simulink model "PID_control"  (R2022a)
settings: Solver=ode3  StartTime=0.0  StopTime=inf  FixedStep=0.005  RelTol=1e-3
undefined symbols (not defined in the file): Angular, Linear
libraries: robotlib x7, robotcorelib x1
settings Model: Creator=Ronak Jain  LastModifiedBy=Ronak Jain
settings OptimizationCC: EnhancedBackFolding=on  PassReuseOutputArgsAs=Individual arguments  LifeSpan=inf  MaxStackSize=64  OptimizeBlockOrder=speed  DifferentSizesBufferReuse=on  OptimizationCustomize=off  EfficientTunableParamExpr=on
settings DebuggingCC: ParameterTunabilityLossMsg=error  BusObjectLabelMismatch=error
settings HardwareCC: ProdBitPerPointer=32  ProdBitPerSizeT=32  ProdBitPerPtrDiffT=32  ProdLargestAtomicFloat=None  ProdIntDivRoundTo=Undefined  ProdEndianess=Unspecified  ProdWordSize=32  ProdHWDeviceType=Generic->Unspecified (assume 32-bit Generic)  TargetBitPerPointer=64  TargetBitPerSizeT=64  TargetBitPerPtrDiffT=64  TargetLongLongMode=on  TargetIntDivRoundTo=Zero  TargetEndianess=LittleEndian  TargetWordSize=64  TargetHWDeviceType=MATLAB Host  ProdEqTarget=off
settings RTWCC: SystemTargetFile=ert.tlc  HardwareBoard=Robot Operating System (ROS)  TLCOptions="-aInlineSetEventsForThisBaseRateFcn=TLC_FALSE -aSuppressMultiTaskScheduler=TLC_FALSE  -aRateBasedStepFcn=0"  TemplateMakefile=ert_default_tmf  Toolchain=Catkin  TargetLang=C++
settings CodeAppCC: ForceParamTrailComments=on  IgnoreCustomStorageClasses=off  OperatorAnnotations=on  SimulinkDataObjDesc=on  SFDataObjDesc=on  InsertBlockDesc=on
settings ERTTargetCC: CodeInterfacePackaging=Reusable function  SupportContinuousTime=on  SupportVariableSizeSignals=on  ModelStepFunctionPrototypeControlCompliant=off  GenerateAllocFcn=on  MultiInstanceErrorCode=None  RootIOFormat=Part of model data structure

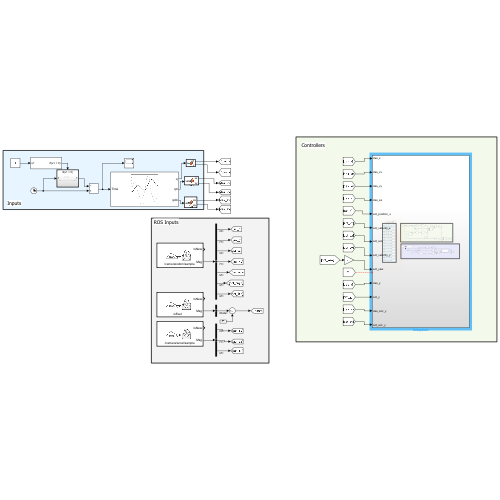
[thumbnail: Simulink's stored preview of the top-level diagram]
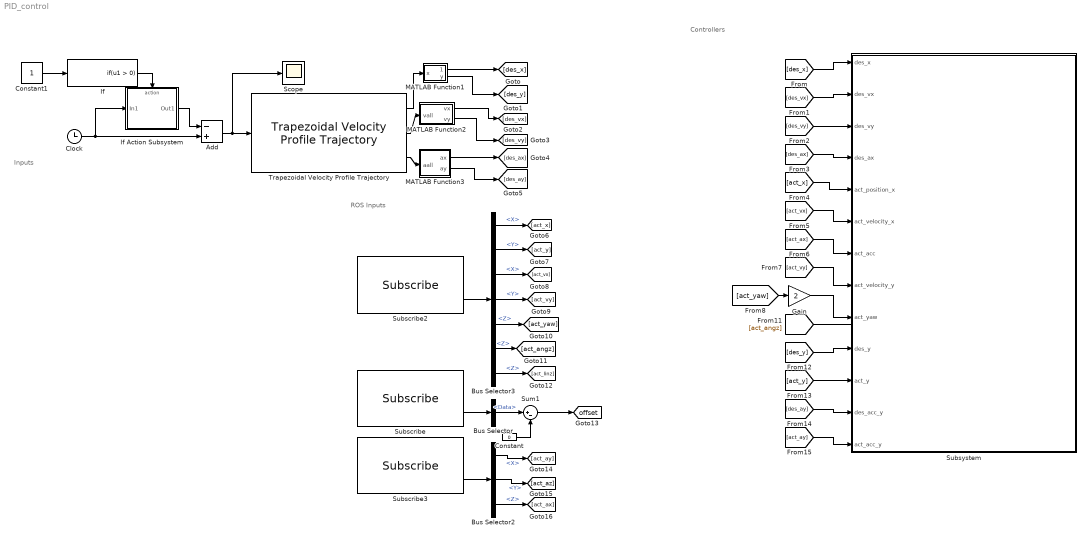
== system PID_control ==
  note: Inputs
  note: ROS Inputs
  note: Controllers
  Add : Sum  Inputs=-+
  Bus Selector : BusSelector  OutputSignals=Data
  Bus Selector2 : BusSelector  OutputSignals=LinearAcceleration.X,LinearAcceleration.Y,LinearAcceleration.Z
  Bus Selector3 : BusSelector  OutputSignals=Pose.Pose.Position.X,Pose.Pose.Position.Y,Twist.Twist.Linear.X,Twist.Twist.Linear.Y,Pose.Pose.Orientation.Z,Twist.Twist.Angular.Z,Twist.Twist.Linear.Z
  Clock : Clock
  Constant : Constant  Value=0
  Constant1 : Constant  SampleTime=-1
  Gain : Gain  Gain=2
  If : If  ShowElse=off
  If Action Subsystem : Subsystem  TreatAsAtomicUnit=on
  MATLAB Function1 : MATLAB Function  TreatAsAtomicUnit=on
  MATLAB Function2 : MATLAB Function  TreatAsAtomicUnit=on
  MATLAB Function3 : MATLAB Function  TreatAsAtomicUnit=on
  Scope : Scope
  Subscribe : robotlib/Subscribe  topicSource=Select from ROS network  topic=/offset  messageType=std_msgs/Float32  SampleTime=-1  legacyBusStruct=off  messageQueueLength=1
  Subscribe2 : robotlib/Subscribe  topicSource=Select from ROS network  topic=/camera/odom/sample  messageType=nav_msgs/Odometry  SampleTime=-1  legacyBusStruct=off  messageQueueLength=1
  Subscribe3 : robotlib/Subscribe  topicSource=Select from ROS network  topic=/camera/accel/sample  messageType=sensor_msgs/Imu  SampleTime=-1  legacyBusStruct=off  messageQueueLength=1
  Subsystem : Subsystem
  Sum1 : Sum  Inputs=|+-
  Trapezoidal Velocity Profile Trajectory : robotcorelib/Trapezoidal Velocity Profile Trajectory  WaypointSource=Internal  Waypoints=[0,2.5*3;0,0]  NumParams=2  Parameter1=Acceleration Time  Parameter2=End Time  ParameterSource=Internal  PeakVelocity=[ 2; 2 ]  Acceleration=[ 1; 2 ]  EndTime=[ 35*3;35*3]  AccelTime=[ 10; 10 ]  SimulateUsing=Interpreted execution
      settings: SourceProductBaseCode=RO,NV,RR,UV
  tag scope: offset=global
  wires:
  Subscribe3/2 -> Bus Selector2/1
  Trapezoidal Velocity Profile Trajectory/1 -> MATLAB Function1/1(x)
  If Action Subsystem/1(Out1) -> Add/1
  Subscribe2/2 -> Bus Selector3/1
  Subscribe/2 -> Bus Selector/1
  If/1 -> If Action Subsystem/Action
  Trapezoidal Velocity Profile Trajectory/2 -> MATLAB Function2/1(vall)
  Trapezoidal Velocity Profile Trajectory/3 -> MATLAB Function3/1(aall)
  Constant1/1 -> If/1
  Clock/1 -> Add/2, If Action Subsystem/1(In1)
  Add/1 -> Scope/1, Trapezoidal Velocity Profile Trajectory/1
  MATLAB Function1/1(x1) -> [des_x]
  MATLAB Function1/2(y) -> [des_y]
  MATLAB Function2/1(vx) -> [des_vx]
  MATLAB Function2/2(vy) -> [des_vy]
  MATLAB Function3/1(ax) -> [des_ax]
  MATLAB Function3/2(ay) -> [des_ay]
  Bus Selector3/1 -> [act_x]  "<X>"
  Bus Selector3/2 -> [act_y]  "<Y>"
  Bus Selector3/3 -> [act_vx]  "<X>"
  Bus Selector3/4 -> [act_vy]  "<Y>"
  Bus Selector3/5 -> [act_yaw]  "<Z>"
  Bus Selector3/6 -> [act_angz]  "<Z>"
  Bus Selector3/7 -> [act_linz]  "<Z>"
  Bus Selector2/1 -> [act_ay]  "<X>"
  Bus Selector2/2 -> [act_az]  "<Y>"
  Bus Selector2/3 -> [act_ax]  "<Z>"
  [des_x] -> Subsystem/1(des_x)
  [des_vx] -> Subsystem/2(des_vx)
  [des_vy] -> Subsystem/3(des_vy)
  [des_ax] -> Subsystem/4(des_ax)
  [act_x] -> Subsystem/5(act_position_x)
  [act_vx] -> Subsystem/6(act_velocity_x)
  [act_ax] -> Subsystem/7(act_acc)
  [act_vy] -> Subsystem/8(act_velocity_y)
  [act_yaw] -> Gain/1
  [act_angz] -> ?
  [des_y] -> Subsystem/10(des_y)
  [act_y] -> Subsystem/11(act_y)
  [des_ay] -> Subsystem/12(des_acc_y)
  [act_ay] -> Subsystem/13(act_acc_y)
  Gain/1 -> Subsystem/9(act_yaw)
  Bus Selector/1 -> Sum1/1  "<Data>"
  Sum1/1 -> [offset]
  Constant/1 -> Sum1/2

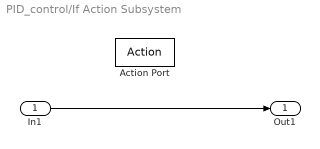
== system PID_control/If Action Subsystem ==
  In1 : Inport
  Action Port : ActionPort  PropagateVarSize=During execution  ActionPortLabel=if(u1 > 0)
  Out1 : Outport
  wires:
  In1/1 -> Out1/1

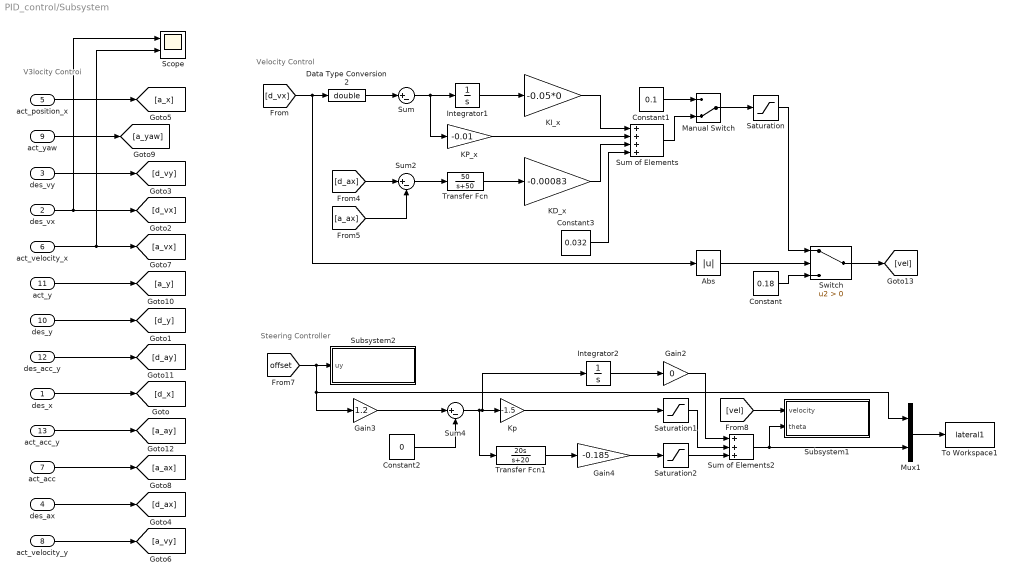
== system PID_control/Subsystem ==
  note: Velocity Control
  note: V3locity Controi
  note: Steering Controller
  des_x : Inport
  des_vx : Inport  Port=2
  des_vy : Inport  Port=3
  des_ax : Inport  Port=4
  act_position_x : Inport  Port=5
  act_velocity_x : Inport  Port=6
  act_acc : Inport  Port=7
  act_velocity_y : Inport  Port=8
  act_yaw : Inport  Port=9
  des_y : Inport  Port=10
  act_y : Inport  Port=11
  des_acc_y : Inport  Port=12
  act_acc_y : Inport  Port=13
  Abs : Abs  SaturateOnIntegerOverflow=off
  Constant : Constant  Value=0.18
  Constant1 : Constant  Value=0.1
  Constant2 : Constant  Value=0
  Constant3 : Constant  Value=0.032
  Data Type Conversion2 : DataTypeConversion  OutDataTypeStr=double  SaturateOnIntegerOverflow=off  RndMeth=Floor
  Gain2 : Gain  Gain=0
  Gain3 : Gain  Gain=1.2
  Gain4 : Gain  Gain=-0.185
  Integrator1 : Integrator
  Integrator2 : Integrator
  KD_x : Gain  Gain=-0.00083
  KI_x : Gain  Gain=-0.05*0
  KP_x : Gain  Gain=-0.01
  Kp : Gain  Gain=-1.5
  Manual Switch : ManualSwitch  CurrentSetting=0
  Mux1 : Mux  Inputs=2
  Saturation : Saturate  LowerLimit=-0.2
  Saturation1 : Saturate  UpperLimit=0.7  LowerLimit=-0.7
  Saturation2 : Saturate  UpperLimit=0.7  LowerLimit=-0.7
  Scope : Scope  NumInputPorts=2
  Subsystem1 : Subsystem
  Subsystem2 : Subsystem
  Sum : Sum  Inputs=|+-
  Sum of Elements : Sum  Inputs=++++
  Sum of Elements2 : Sum  Inputs=+++
  Sum2 : Sum  Inputs=|+-
  Sum4 : Sum  Inputs=|+-
  Switch : Switch  Criteria=u2 > Threshold  SaturateOnIntegerOverflow=off  InputSameDT=off
  To Workspace1 : ToWorkspace  VariableName=lateral1  SaveFormat=Timeseries  SampleTime=-1
  Transfer Fcn : TransferFcn  Numerator=[50]  Denominator=[1 50]
  Transfer Fcn1 : TransferFcn  Numerator=[20 0]  Denominator=[1 20]
  wires:
  KD_x/1 -> Sum of Elements/3
  Abs/1 -> Switch/2
  des_vx/1 -> Scope/1, [d_vx]
  des_vy/1 -> [d_vy]
  Constant/1 -> Switch/3
  Transfer Fcn/1 -> KD_x/1
  Manual Switch/1 -> Saturation/1
  Switch/1 -> [vel]
  Sum of Elements/1 -> Manual Switch/2
  Saturation/1 -> Switch/1
  Constant1/1 -> Manual Switch/1
  Constant3/1 -> Sum of Elements/4
  [a_ax] -> Sum2/2
  [d_ax] -> Sum2/1
  Sum2/1 -> Transfer Fcn/1
  KI_x/1 -> Sum of Elements/1
  Integrator1/1 -> KI_x/1
  act_velocity_y/1 -> [a_vy]
  act_yaw/1 -> [a_yaw]
  KP_x/1 -> Sum of Elements/2
  Data Type Conversion2/1 -> Sum/1
  Sum/1 -> KP_x/1, Integrator1/1
  des_x/1 -> [d_x]
  [d_vx] -> Data Type Conversion2/1, Abs/1
  des_acc_y/1 -> [d_ay]
  act_acc_y/1 -> [a_ay]
  des_y/1 -> [d_y]
  act_y/1 -> [a_y]
  act_velocity_x/1 -> Scope/2, [a_vx]
  act_acc/1 -> [a_ax]
  des_ax/1 -> [d_ax]
  act_position_x/1 -> [a_x]
  [offset] -> Mux1/1, Gain3/1, Subsystem2/1(uy)
  Gain2/1 -> Sum of Elements2/1
  Sum4/1 -> Kp/1, Integrator2/1, Transfer Fcn1/1
  [vel] -> Subsystem1/1(velocity)
  Sum of Elements2/1 -> Mux1/2, Subsystem1/2(theta)
  Constant2/1 -> Sum4/2
  Transfer Fcn1/1 -> Gain4/1
  Saturation1/1 -> Sum of Elements2/2
  Mux1/1 -> To Workspace1/1
  Integrator2/1 -> Gain2/1
  Gain3/1 -> Sum4/1
  Saturation2/1 -> Sum of Elements2/3
  Kp/1 -> Saturation1/1
  Gain4/1 -> Saturation2/1

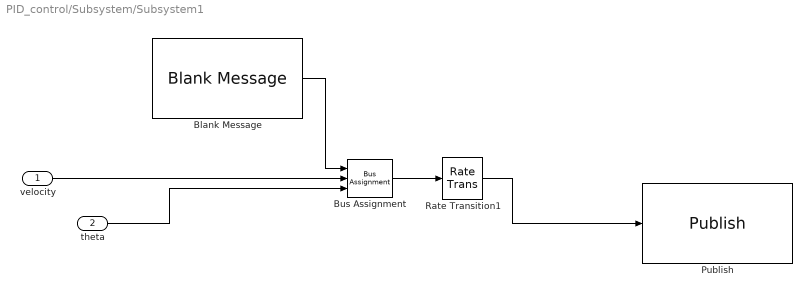
== system PID_control/Subsystem/Subsystem1 ==
  velocity : Inport
  theta : Inport  Port=2
  Blank Message : robotlib/Blank Message  messageClass=Message  entityType=geometry_msgs/Twist  messageType=geometry_msgs/Twist  SampleTime=-1  legacyBusStruct=off
  Bus Assignment : BusAssignment  AssignedSignals=Linear.X,Angular.Z
  Publish : robotlib/Publish  topicSource=Specify your own  topic=/move_velocity  messageType=geometry_msgs/Twist  legacyBusStruct=off  messageQueueLength=1
  Rate Transition1 : RateTransition
  wires:
  theta/1 -> Bus Assignment/3
  Blank Message/1 -> Bus Assignment/1
  Bus Assignment/1 -> Rate Transition1/1
  velocity/1 -> Bus Assignment/2
  Rate Transition1/1 -> Publish/1

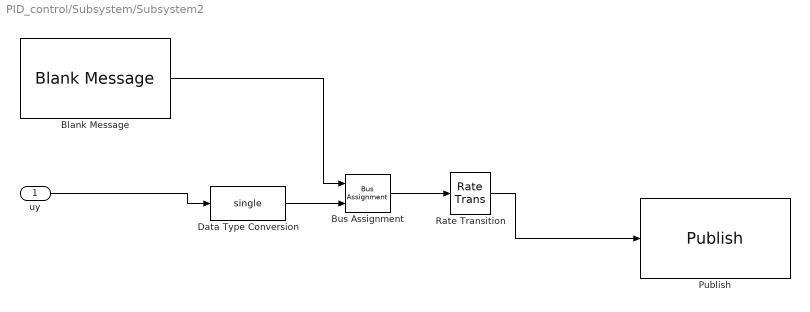
== system PID_control/Subsystem/Subsystem2 ==
  uy : Inport
  Blank Message : robotlib/Blank Message  messageClass=Message  entityType=std_msgs/Float32  messageType=std_msgs/Float32  SampleTime=-1  legacyBusStruct=off
  Bus Assignment : BusAssignment  AssignedSignals=Data
  Data Type Conversion : DataTypeConversion  OutDataTypeStr=single  SaturateOnIntegerOverflow=off  RndMeth=Floor
  Publish : robotlib/Publish  topicSource=Specify your own  topic=/uy  messageType=std_msgs/Float32  legacyBusStruct=off  messageQueueLength=1
  Rate Transition : RateTransition
  wires:
  uy/1 -> Data Type Conversion/1
  Bus Assignment/1 -> Rate Transition/1
  Data Type Conversion/1 -> Bus Assignment/2
  Blank Message/1 -> Bus Assignment/1
  Rate Transition/1 -> Publish/1

== matlab function PID_control/MATLAB Function2 ==
  data: vall input; vx output; vy output
function [vx,vy] = fcn(vall)
vx = vall(1,:);
vy = vall(2,:);

== matlab function PID_control/MATLAB Function3 ==
  data: aall input; ax output; ay output
function [ax,ay]  = fcn(aall)
ax = aall(1,:);
ay = aall(2,:);
end

== matlab function PID_control/MATLAB Function1 ==
  data: x1 output; x input; y output
function [x1,y] = fcn(x)

x1 = x(1,:);
y  = x(2,:);

end
